simulink model "house_thermal_model"  (R2019a)
settings: Solver=ode3  StartTime=0.0  StopTime=604800  FixedStep=10  RelTol=1e-3  AbsTol=1e-6
model workspace (MATLAB code in the model file):
  | % load initial conditions and physical properties from file
  | 
  | house_thermal_model_init
values from neighbouring files (symbols this model uses):
  c_a = simdata.Simulation.Material.c_a.value    [house_heat_model_init.m]    (also in house_thermal_model_init.m)
  c_floor = simdata.Simulation.Material.c_floor.value    [house_heat_model_init.m]    (also in house_thermal_model_init.m)
  c_s = simdata.Simulation.Material.c_s.value    [house_heat_model_init.m]    (also in house_thermal_model_init.m)
  c_water = simdata.Simulation.Material.c_water.value    [house_heat_model_init.m]    (also in house_thermal_model_init.m)
  dt = simdata.Simulation.dt.value    [control_sim.m]    (also in house_heat_model_init.m; house_thermal_model_init.m)
  dT_histerezis = simdata.Simulation.Heat.dT_histerizes.value    [house_heat_model_init.m]    (also in house_thermal_model_init.m)
  M_air = (lenHouse*widHouse*htHouse+tan(pitRoof)*widHouse*lenHouse)*densAir    [house_heat_model_init.m]    (also in house_thermal_model_init.m)
  M_floor = floorArea*L_floor*densConcrete*heatedPct    [house_heat_model_init.m]    (also in house_thermal_model_init.m)
  Mdot = simdata.Simulation.Heat.M_dot.value    [house_heat_model_init.m]    (also in house_thermal_model_init.m)
  R_floor = L_floor/(k_floor*floorArea)    [house_heat_model_init.m]    (also in house_thermal_model_init.m)
  R_house = R_wall*R_window/(R_wall + R_window)    [house_heat_model_init.m]    (also in house_thermal_model_init.m)
  T_pred = y_pred    [control_sim.m]    (also in house_thermal_model_init.m = single(0))
  THeater = simdata.Simulation.Heat.T_Heater.value    [house_heat_model_init.m]    (also in house_thermal_model_init.m)
  TinIC = simdata.Simulation.Heat.T_IN_ini.value    [house_heat_model_init.m]    (also in house_thermal_model_init.m)
libraries: simulink x2, dspswit3 x1
settings Model: ExtModeTrigMode=oneshot  ExtModeArmWhenConnect=off  ExtModeAutoUpdateStatusClock=off  OrderedModelArguments=off  Creator=The MathWorks Inc.  LastModifiedBy=szabo
settings SolverCC: AutoScaleAbsTol=off
settings DataIOCC: Decimation=5  ExternalInput=[]  InitialState=[]  SaveFormat=Array  SaveOutput=off  SignalLogging=off  SaveTime=off  ReturnWorkspaceOutputs=off  SignalLoggingName=sldemo_househeat_output
settings OptimizationCC: BlockReduction=off  BooleanDataType=off  ExpressionDepthLimit=2147483647  InitFltsAndDblsToZero=on  LifeSpan=inf  BufferReusableBoundary=off
settings DebuggingCC: SaveWithParameterizedLinksMsg=none  UnderspecifiedInitializationDetection=Classic  MergeDetectMultiDrivingBlocksExec=none  SignalResolutionControl=TryResolveAllWithWarning  MultiTaskDSMMsg=warning  MultiTaskCondExecSysMsg=none  IntegerOverflowMsg=none  FcnCallInpInsideContextMsg=warning  BusObjectLabelMismatch=none  StateNameClashWarn=warning  SFUnexpectedBacktrackingDiag=warning  SFNoUnconditionalDefaultTransitionDiag=warning  SFExecutionAtInitializationDiag=none  IntegerSaturationMsg=none  ArithmeticOperatorsInVariantConditions=warning
settings HardwareCC: ProdBitPerPointer=32  ProdBitPerSizeT=32  ProdBitPerPtrDiffT=32  ProdLargestAtomicFloat=None  ProdIntDivRoundTo=Undefined  ProdEndianess=Unspecified  ProdWordSize=32  ProdHWDeviceType=32-bit Generic  TargetUnknown=on
settings ModelReferenceCC: PropagateSignalLabelsOutOfModel=off
settings SFSimCC: SimUseLocalCustomCode=off
settings RTWCC: Description=Generic Real-Time Target  RTWUseLocalCustomCode=off
settings CodeAppCC: StateflowObjectComments=on
settings GRTTargetCC: TargetFcnLib=ansi_tfl_tmw.mat  TargetLangStandard=C89/C90 (ANSI)  GeneratePreprocessorConditionals=Disable all  CombineOutputUpdateFcns=off  GRTInterface=on
settings ConfigComp: CovMetricSettings=dw  CovHtmlReporting=on  CovSaveCumulativeToWorkspaceVar=on  CovSaveSingleToWorkspaceVar=on  CovExternalEMLEnable=off  CovSFcnEnable=off
settings SimscapeCC: SimscapeNormalizeSystem=off

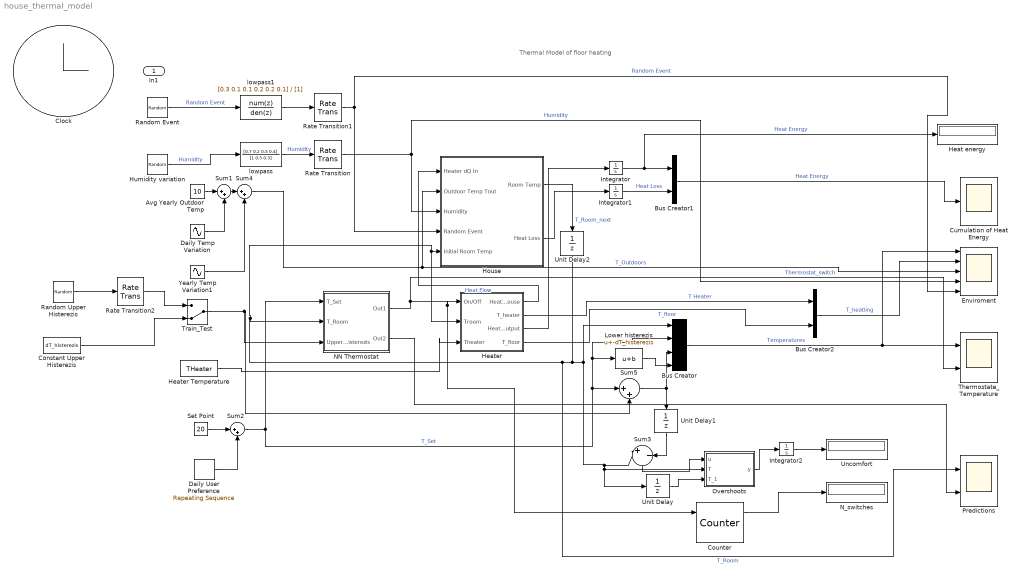
== system house_thermal_model ==
  note: Thermal Model of floor heating
  In1 : Inport
  Avg Yearly Outdoor Temp : Constant  Value=10
  Bus Creator : BusCreator  Inputs=4
  Bus Creator1 : BusCreator  Inputs=2
  Bus Creator2 : BusCreator  Inputs=2
  Clock : Clock
  Constant Upper Histerezis : Constant  Value=dT_histerezis  SampleTime=dt
  Counter : dspswit3/Counter  Direction=Up  CountEvent=Rising edge  CounterSize=32 bits  MaxCount=255  InitialCount=0  Output=Count and Hit  HitValue=32  ResetInput=on  SamplesPerFrame=1  Ts=1  CntDtype=double  HitDtype=Logical
  Cumulation of Heat Energy : Scope
  Daily Temp Variation : Sin  Amplitude=5  Frequency=2*pi/(24*3600)  SampleTime=dt
  Daily User Preference : simulink/Sources/Repeating Sequence  rep_seq_t=[0 25199 25200 32399 32400 57599 57600 79199 79200]  rep_seq_y=[-1 -1 1 1 -2 -2 1 1 -1]
  Enviroment : Scope  NumInputPorts=5
  Heat energy : Display
  Heater : Subsystem
      settings: MinAlgLoopOccurrences=on
      mask Display: image('D:\Projects\ThermoNN\misc\Heater.png');
  Heater Temperature : Constant  Value=THeater
  House : Subsystem
      settings: MinAlgLoopOccurrences=on
      mask Display: image('D:\Projects\ThermoNN\misc\House.png');
  Humidity variation : RandomNumber  Description=Random events in heat capacity of the room - like window opening, persons in the house, e.t.c  Mean=0.7  Variance=0.05  SampleTime=3600*24
  Integrator : Integrator
  Integrator1 : Integrator
  Integrator2 : Integrator
  Lower histerezis : Bias  Bias=-dT_histerezis
  "NN Thermostat " : Subsystem
      settings: MinAlgLoopOccurrences=on
      mask Display: image('D:\Projects\ThermoNN\misc\Thermostate.png');
  N_switches : Display
  Overshoots : MATLAB Function  TreatAsAtomicUnit=on
  Predictions : Scope  NumInputPorts=2
  Random Event : RandomNumber  Mean=1.2  Variance=0.01  SampleTime=3600
  Random Upper Histerezis : UniformRandomNumber  Minimum=0  Maximum=dT_histerezis  SampleTime=3600
  Rate Transition : RateTransition  InitialCondition=0.7
  Rate Transition1 : RateTransition  InitialCondition=1
  Rate Transition2 : RateTransition  InitialCondition=0.25
  Set Point : Constant  Value=20
  Sum{1..2,4..5} (4 alike) : Sum  Inputs=|++  SaturateOnIntegerOverflow=on  InputSameDT=on  OutDataTypeStr=Inherit: Same as first input
  Sum3 : Sum  Inputs=|+||-  SaturateOnIntegerOverflow=on  InputSameDT=on  OutDataTypeStr=Inherit: Same as first input
  Thermostate_Temperature : Scope  NumInputPorts=2
  Train_Test : ManualSwitch  CurrentSetting=0
  Uncomfort : Display
  Unit Delay : UnitDelay  InitialCondition=TinIC  SampleTime=-1  HasFrameUpgradeWarning=on
  Unit Delay1 : UnitDelay  InitialCondition=TinIC  SampleTime=-1  HasFrameUpgradeWarning=on
  Unit Delay2 : UnitDelay  InitialCondition=TinIC  SampleTime=-1  HasFrameUpgradeWarning=on
  Yearly Temp Variation1 : Sin  Amplitude=10  Frequency=2*pi/(365*24*3600)  Phase=-3*pi/4  SampleTime=dt
  lowpass : DiscreteFilter  Numerator=[0.7 0.2 0.5 0.4]  Denominator=[1 0.5 0.3]  InitialStates=0.5  SampleTime=3600  a0EqualsOne=on
  lowpass1 : DiscreteFilter  Numerator=[0.3 0.1 0.1 0.2 0.2 0.1]  Denominator=[1]  InitialStates=1  SampleTime=120  a0EqualsOne=on
  wires:
  Integrator/1 -> Heat energy/1, Bus Creator1/1  "Heat Energy"
  Daily Temp Variation/1 -> Sum1/2
  Sum4/1 -> Enviroment/3, House/2(Outdoor Temp Tout)  "T_Outdoors"
  Avg Yearly Outdoor Temp/1 -> Sum1/1
  House/1("Room Temp ") -> Unit Delay2/1  "T_Room_next"
  Heater/1("HeatFlowToHouse ") -> House/1(Heater dQ In)  "Heat Flow"
  Daily User Preference/1 -> Sum2/2
  Set Point/1 -> Sum2/1
  Sum2/1 -> "NN Thermostat "/1(T_Set), Sum5/1, Lower histerezis/1, Bus Creator/2  "T_Set"
  Bus Creator/1 -> Enviroment/1, Thermostate_Temperature/1  "Temperatures"
  Sum5/1 -> Bus Creator/3, Unit Delay1/1
  Random Event/1 -> lowpass1/1  "Random Event"
  Heater/3(HeaterOutput) -> Integrator/1
  House/2(Heat Loss) -> Integrator1/1
  Integrator1/1 -> Bus Creator1/2  "Heat Loss"
  Overshoots/1(y) -> Integrator2/1
  Integrator2/1 -> Uncomfort/1
  Counter/1 -> N_switches/1
  Humidity variation/1 -> lowpass/1  "Humidity"
  lowpass/1 -> Rate Transition/1  "Humidity"
  lowpass1/1 -> Rate Transition1/1
  "NN Thermostat "/1(Out1) -> Thermostate_Temperature/2, Counter/1, Heater/1(On/Off)  "Thermostat_switch"
  Unit Delay2/1 -> Predictions/1, House/5("Initial Room Temp "), Heater/2(Troom), "NN Thermostat "/2(T_Room), Bus Creator/1, Sum3/1, Overshoots/2(T), Unit Delay/1  "T_Room"
  Sum3/1 -> Overshoots/1(u)
  Unit Delay/1 -> Overshoots/3(T_1)
  Unit Delay1/1 -> Sum3/2
  Lower histerezis/1 -> Bus Creator/4
  "NN Thermostat "/2(Out2) -> Predictions/2
  Rate Transition/1 -> House/3(Humidity), Enviroment/4  "Humidity"
  Rate Transition1/1 -> House/4("Random Event "), Enviroment/5  "Random Event"
  Heater Temperature/1 -> Heater/3(Theater)
  Sum1/1 -> Sum4/1
  Yearly Temp Variation1/1 -> Sum4/2
  Bus Creator2/1 -> Enviroment/2  "T_heatiing"
  Heater/2("T_heater ") -> Bus Creator2/1  "T Heater"
  Heater/4(T_floor) -> Bus Creator2/2  "T_floor"
  Random Upper Histerezis/1 -> Rate Transition2/1
  Train_Test/1 -> Sum5/2, "NN Thermostat "/3(Upper Histerezis)
  Constant Upper Histerezis/1 -> Train_Test/2
  Rate Transition2/1 -> Train_Test/1
  Bus Creator1/1 -> Cumulation of Heat Energy/1  "Heat Energy"

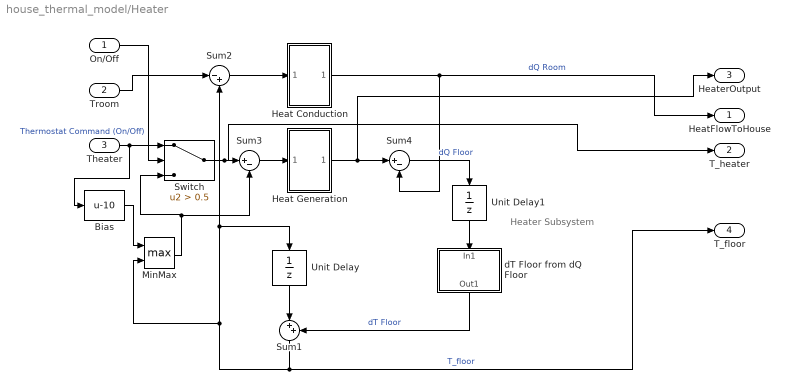
== system house_thermal_model/Heater ==
  note: Heater Subsystem
  On/Off : Inport
  Troom : Inport  Port=2
  Theater : Inport  Port=3
  Bias : Bias  Bias=-10
  Heat Generation : Subsystem  Description=assumption: all heater energy is transmitted to the floor and house heating
  Heat Conduction : Subsystem
  MinMax : MinMax  Function=max  Inputs=2
  Sum1 : Sum  Inputs=|++
  Sum2 : Sum  Inputs=|-+
  Sum3 : Sum  Inputs=|+-
  Sum4 : Sum  Inputs=|+-
  Switch : Switch  Criteria=u2 > Threshold  Threshold=0.5
  Unit Delay : UnitDelay  InitialCondition=TinIC  SampleTime=-1  HasFrameUpgradeWarning=on
  Unit Delay1 : UnitDelay  InitialCondition=TinIC  SampleTime=-1  HasFrameUpgradeWarning=on
  dT Floor from dQ Floor : Subsystem
  "HeatFlowToHouse " : Outport
  "T_heater " : Outport  Port=2
  HeaterOutput : Outport  Port=3
  T_floor : Outport  Port=4
  wires:
  Troom/1 -> Sum2/1
  Sum2/1 -> Heat Conduction/1(In1)
  On/Off/1 -> Switch/2  "Thermostat Command (On/Off)"
  Unit Delay/1 -> Sum1/1
  Sum1/1 -> MinMax/2, Sum2/2, Unit Delay/1, T_floor/1  "T_floor"
  Theater/1 -> Bias/1, Switch/1
  dT Floor from dQ Floor/1(Out1) -> Sum1/2  "dT Floor"
  Heat Conduction/1(Out1) -> "HeatFlowToHouse "/1, Sum4/2  "dQ Room"
  Switch/1 -> "T_heater "/1, Sum3/1
  Sum3/1 -> Heat Generation/1(In1)
  Heat Generation/1(Out1) -> HeaterOutput/1, Sum4/1
  Sum4/1 -> Unit Delay1/1  "dQ Floor"
  Unit Delay1/1 -> dT Floor from dQ Floor/1(In1)
  Bias/1 -> MinMax/1
  MinMax/1 -> Sum3/2, Switch/3

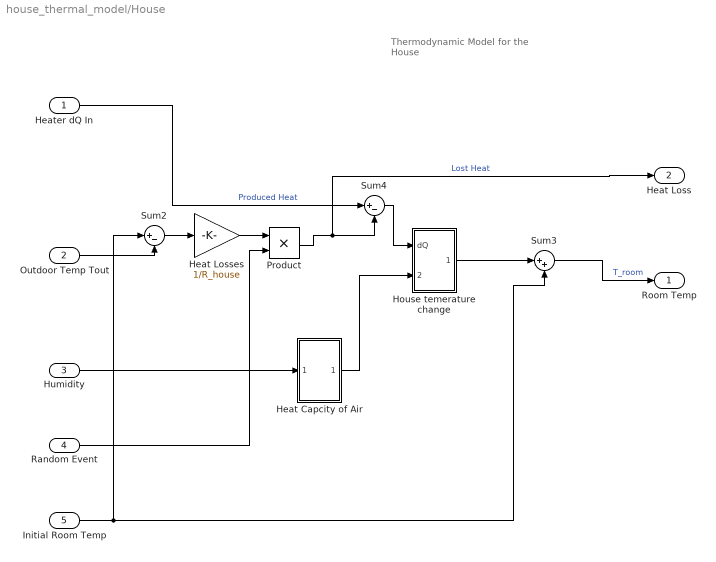
== system house_thermal_model/House ==
  note: Thermodynamic Model
      | for the House
  Heater dQ In : Inport
  Outdoor Temp Tout : Inport  Port=2
  Humidity : Inport  Port=3
  "Random Event " : Inport  Port=4
  "Initial Room Temp " : Inport  Port=5
  "Heat Capcity of Air " : Subsystem
  Heat Losses : Gain  Gain=1/R_house  SaturateOnIntegerOverflow=on  OutDataTypeStr=Inherit: Same as input  ParamDataTypeStr=Inherit: Same as input
  House temerature change : Subsystem
  Product : Product
  Sum2 : Sum  Inputs=|+-  SaturateOnIntegerOverflow=on  InputSameDT=on  OutDataTypeStr=Inherit: Same as first input
  Sum3 : Sum  Inputs=|++
  Sum4 : Sum  Inputs=|+-  SaturateOnIntegerOverflow=on  InputSameDT=on  OutDataTypeStr=Inherit: Same as first input
  "Room Temp " : Outport  InitialOutput=0
  Heat Loss : Outport  Port=2  InitialOutput=0
  wires:
  Outdoor Temp Tout/1 -> Sum2/2
  Sum2/1 -> Heat Losses/1
  Sum3/1 -> "Room Temp "/1  "T_room"
  Heater dQ In/1 -> Sum4/1  "Produced Heat"
  House temerature change/1(Out1) -> Sum3/1
  Sum4/1 -> House temerature change/1(dQ)
  Humidity/1 -> "Heat Capcity of Air "/1(In1)
  "Heat Capcity of Air "/1(Out1) -> House temerature change/2(Heat Capacity)
  "Random Event "/1 -> Product/2
  Heat Losses/1 -> Product/1
  Product/1 -> Heat Loss/1, Sum4/2  "Lost Heat"
  "Initial Room Temp "/1 -> Sum2/1, Sum3/2

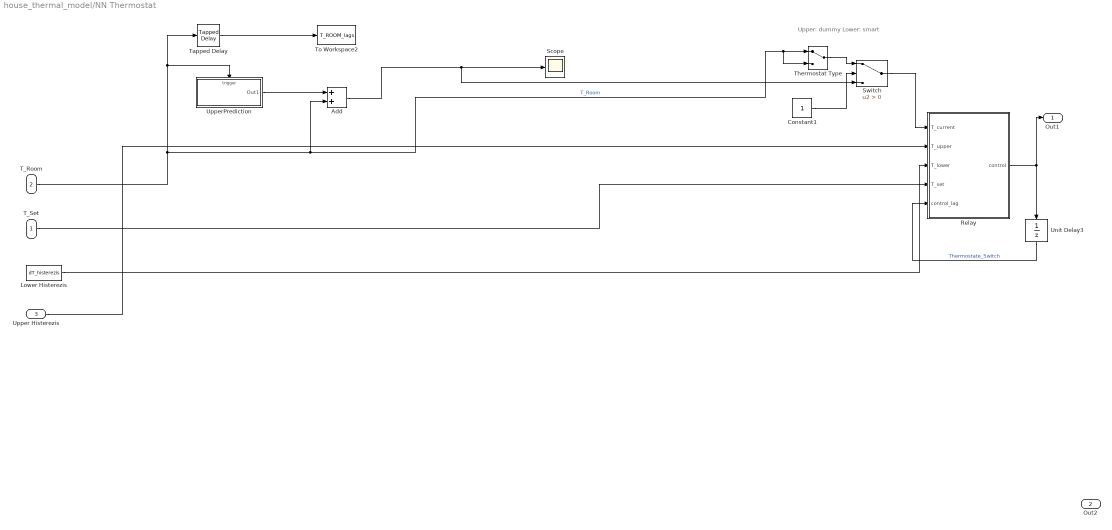
== system house_thermal_model/NN Thermostat  ==
  note: Upper: dummy
      | Lower: smart
  T_Set : Inport
  T_Room : Inport  Port=2
  Upper Histerezis : Inport  Port=3
  Add : Sum
  Constant1 : Constant
  Lower Histerezis : Constant  Value=dT_histerezis
  Relay : MATLAB Function  TreatAsAtomicUnit=on
  Scope : Scope
  Switch : Switch  Criteria=u2 > Threshold
  Tapped Delay : simulink/Discrete/Tapped Delay  vinit=TinIC  samptime=-1  NumDelays=25  DelayOrder=Oldest  includeCurrent=off
  Thermostat Type : ManualSwitch  Description=|
      | Turn on/off smart thermostat
      | Off: Up
      | On: Down
  To Workspace2 : ToWorkspace  VariableName=T_ROOM_lags  SaveFormat=Timeseries  SampleTime=-1
      settings: MaxDataPoints=1
  Unit Delay3 : UnitDelay  SampleTime=-1  HasFrameUpgradeWarning=on
  UpperPrediction : Subsystem  TreatAsAtomicUnit=on
  Out1 : Outport
  Out2 : Outport  Port=2
  wires:
  Relay/1(control) -> Out1/1, Unit Delay3/1
  Switch/1 -> Relay/1(T_current)
  Unit Delay3/1 -> Relay/5(control_lag)  "Thermostate_Switch"
  Thermostat Type/1 -> Switch/1
  T_Room/1 -> Add/2, Thermostat Type/2, Thermostat Type/1, UpperPrediction/Trigger, Tapped Delay/1  "T_Room"
  T_Set/1 -> Relay/4(T_set)
  Lower Histerezis/1 -> Relay/3(T_lower)
  Upper Histerezis/1 -> Relay/2(T_upper)
  Tapped Delay/1 -> To Workspace2/1
  Constant1/1 -> Switch/2
  UpperPrediction/1(Out1) -> Add/1
  Add/1 -> Switch/3, Scope/1

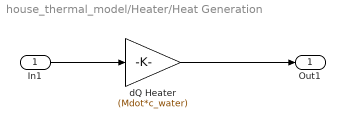
== system house_thermal_model/Heater/Heat Generation ==
  In1 : Inport
  dQ Heater : Gain  Gain=(Mdot*c_water)
  Out1 : Outport
  wires:
  In1/1 -> dQ Heater/1
  dQ Heater/1 -> Out1/1

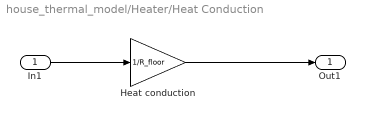
== system house_thermal_model/Heater/Heat Conduction ==
  In1 : Inport
  Heat conduction : Gain  Gain=1/R_floor
  Out1 : Outport
  wires:
  In1/1 -> Heat conduction/1
  Heat conduction/1 -> Out1/1

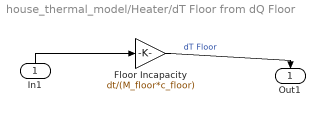
== system house_thermal_model/Heater/dT Floor from dQ Floor ==
  In1 : Inport
  Floor Incapacity : Gain  Gain=dt/(M_floor*c_floor)
  Out1 : Outport
  wires:
  In1/1 -> Floor Incapacity/1
  Floor Incapacity/1 -> Out1/1  "dT Floor"

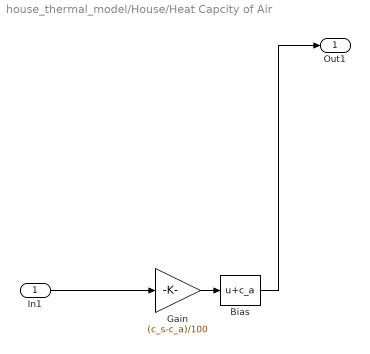
== system house_thermal_model/House/Heat Capcity of Air  ==
  In1 : Inport
  Bias : Bias  Bias=c_a
  Gain : Gain  Gain=(c_s-c_a)/100  SaturateOnIntegerOverflow=on  OutDataTypeStr=Inherit: Same as input  ParamDataTypeStr=Inherit: Same as input
  Out1 : Outport
  wires:
  In1/1 -> Gain/1
  Bias/1 -> Out1/1
  Gain/1 -> Bias/1

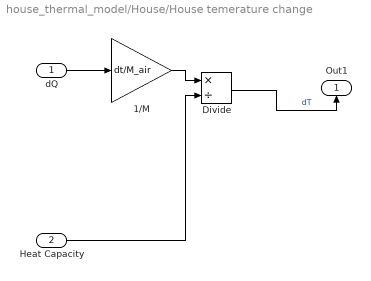
== system house_thermal_model/House/House temerature change ==
  dQ : Inport
  Heat Capacity : Inport  Port=2
  1/M : Gain  Gain=dt/M_air  SaturateOnIntegerOverflow=on  OutDataTypeStr=Inherit: Same as input  ParamDataTypeStr=Inherit: Same as input
  Divide : Product  Inputs=*/
  Out1 : Outport
  wires:
  1/M/1 -> Divide/1
  dQ/1 -> 1/M/1
  Divide/1 -> Out1/1  "dT"
  Heat Capacity/1 -> Divide/2

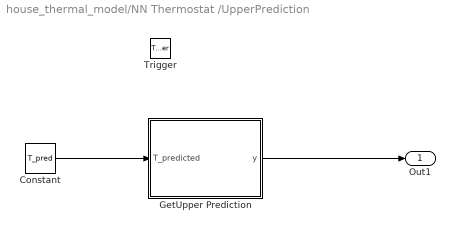
== system house_thermal_model/NN Thermostat /UpperPrediction ==
  Trigger : TriggerPort  VariantControl=Variant
  Constant : Constant  Value=T_pred
  GetUpper Prediction : MATLAB Function  TreatAsAtomicUnit=on
  Out1 : Outport
  wires:
  GetUpper Prediction/1(y) -> Out1/1
  Constant/1 -> GetUpper Prediction/1(T_predicted)

== matlab function house_thermal_model/NN Thermostat /UpperPrediction/GetUpper Prediction ==
  data: y output; T_predicted input
function y = fcn(T_predicted)
y=T_predicted;
coder.extrinsic('evalin')
y = evalin('base','T_pred');

== matlab function house_thermal_model/Overshoots ==
  data: u input; y output; T input; T_1 input
function y = fcn(u,T,T_1)
% overshoots

if (u>0) && (T>T_1)
    % rising temperature
    y=u;
else
    y=0;
end

== matlab function house_thermal_model/NN Thermostat /Relay ==
  data: T_current input; T_upper input; T_lower input; T_set input; control_lag input; control output
function control = fcn(T_current,T_upper,T_lower,T_set,control_lag)
% overshoots

dT=T_set-T_current;

if control_lag==1 
    % heating
    if (-dT>T_upper)
        control=0;
    else
        control=1;
    end
else
    % not heating
    if (dT>T_lower)
        control=1;
    else
        control=0;
    end
end
